simulink model "untitled"  (R2020a)
settings: Solver=VariableStepAuto  StartTime=0.0  StopTime=0.5  RelTol=1e-3
values from neighbouring files (symbols this model uses):
  acc = [3.6 1.8 1.8 1.8 1.8 1.8 -3.6 -7.2 -9 -9 -10.8 -10.8 ... (316 elements, 316x1)]    [workspacecar.mat]
  Crf = 0.015    [Untitled2.m]    (also in workspacecar.mat)
  GVM = 900    [Untitled2.m]    (also in workspacecar.mat)
  GVW = GVM*g    (= 8829)    [Untitled2.m]    (also in workspacecar.mat)
  Rw = 0.2286    [Untitled2.m]    (also in workspacecar.mat)
  totalforce = [13704.43617 12241.1843831 12241.1843831 12399.9815925 12399.9815925 12560.8277981 7700.82779813 4141.18438313 2209.73695313 1757.93328 -153.0241875 -710.3511675 ... (316 elements, 316x1)]    [workspacecar.mat]
  VelocityKmph = [273.6 277.2 277.2 280.8 280.8 284.4 284.4 277.2 270 259.2 252 237.6 ... (316 elements, 316x1)]    [workspacecar.mat]
libraries: simulink_extras x1
settings Model: Creator=Khojasteh Mirza  LastModifiedBy=Khojasteh Mirza

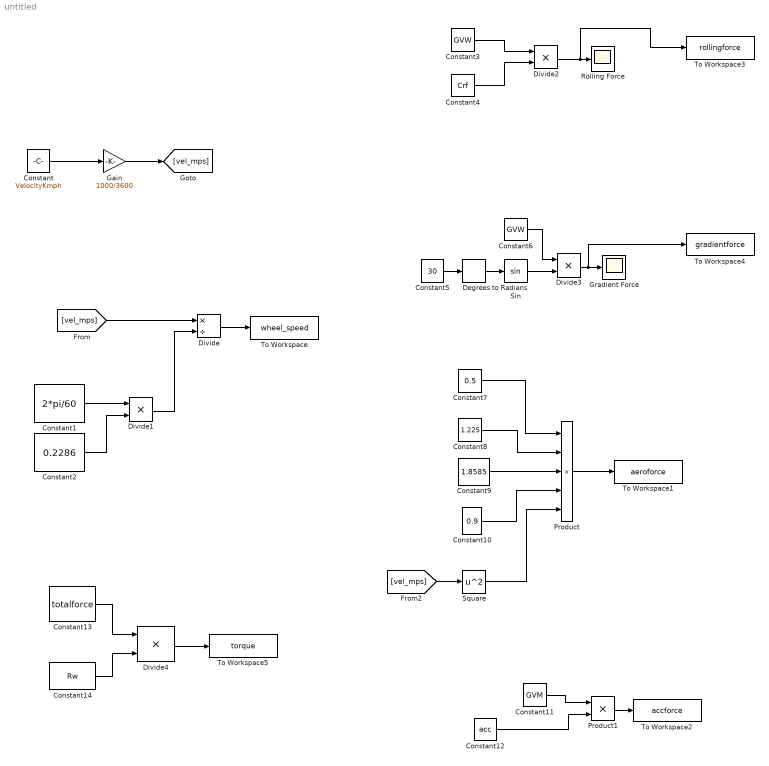
== system untitled ==
  Constant : Constant  Value=VelocityKmph
  Constant1 : Constant  Value=2*pi/60
  Constant10 : Constant  Value=0.9
  Constant11 : Constant  Value=GVM
  Constant12 : Constant  Value=acc
  Constant13 : Constant  Value=totalforce
  Constant14 : Constant  Value=Rw
  Constant2 : Constant  Value=0.2286
  Constant3 : Constant  Value=GVW  SampleTime=-1
  Constant4 : Constant  Value=Crf  SampleTime=-1
  Constant5 : Constant  Value=30  SampleTime=-1
  Constant6 : Constant  Value=GVW  SampleTime=-1
  Constant7 : Constant  Value=0.5
  Constant8 : Constant  Value=1.225
  Constant9 : Constant  Value=1.8585
  Degrees to Radians : simulink_extras/Transformations/Degrees to Radians
  Divide : Product  Inputs=*/
  Divide{1..4} (4 alike) : Product  Inputs=**
  Gain : Gain  Gain=1000/3600
  Gradient Force : Scope
  Product : Product  Inputs=5
  Product1 : Product
  Rolling Force : Scope
  Sin : Trigonometry
  Square : Math  Operator=square  SaturateOnIntegerOverflow=on
  To Workspace : ToWorkspace  VariableName=wheel_speed  SampleTime=-1
  To Workspace1 : ToWorkspace  VariableName=aeroforce  SampleTime=-1
  To Workspace2 : ToWorkspace  VariableName=accforce  SampleTime=-1
  To Workspace3 : ToWorkspace  VariableName=rollingforce  SampleTime=-1
  To Workspace4 : ToWorkspace  VariableName=gradientforce  SampleTime=-1
  To Workspace5 : ToWorkspace  VariableName=torque  SampleTime=-1
  wires:
  Constant/1 -> Gain/1
  Gain/1 -> [vel_mps]
  [vel_mps] -> Divide/1
  Constant1/1 -> Divide1/1
  Constant2/1 -> Divide1/2
  Divide1/1 -> Divide/2
  Divide/1 -> To Workspace/1
  Constant3/1 -> Divide2/1
  Constant4/1 -> Divide2/2
  Divide2/1 -> To Workspace3/1, Rolling Force/1
  Constant5/1 -> Degrees to Radians/1
  Degrees to Radians/1 -> Sin/1
  Sin/1 -> Divide3/2
  Constant6/1 -> Divide3/1
  Divide3/1 -> To Workspace4/1, Gradient Force/1
  [vel_mps] -> Square/1
  Constant9/1 -> Product/3
  Constant8/1 -> Product/2
  Constant10/1 -> Product/4
  Constant7/1 -> Product/1
  Square/1 -> Product/5
  Product/1 -> To Workspace1/1
  Constant12/1 -> Product1/2
  Constant11/1 -> Product1/1
  Product1/1 -> To Workspace2/1
  Constant13/1 -> Divide4/1
  Constant14/1 -> Divide4/2
  Divide4/1 -> To Workspace5/1
